simulink model "friction"  (R2017a)
settings: Solver=ode1  StartTime=0.0  StopTime=50  FixedStep=1e-3  RelTol=1e-3
values from neighbouring files (symbols this model uses):
  ctrl_mass = mass    (= 1)    [Script_Friction.m]
  ctrl_ts = 1e-3    (= 0.001)    [Script_Friction.m]
  Fapp = Fc/2    (= 1.5)    [Script_Friction.m]
  Fc = 2.4    [Script_Friction.m]
  Fs = 4.9    [Script_Friction.m]
  i = 6.7    [Script_Friction.m]
  kv = 40.101e-2    (= 0.40101)    [Script_Friction.m]
  m = 3.14    [Static_Identif.m]    (also in static_optim.m)
  mass = 8.1    [C_script_dyn_optimization.m]    (also in Script_Friction.m = 1; identify_dynamic_param.m)
  N = 100    [A_Static_Experiment.m]    (also in identify_static_param.m; obtain_sim_data.m = round(length(x) / 2); run_sim.m)
  sigma0 = 10e4    (= 100000)    [Script_Friction.m]
  sigma1 = 500    [Script_Friction.m]
  sigma2 = 0.1    [C_script_dyn_optimization.m]    (also in Script_Friction.m = 11.1)
  vs = 1.6e1    (= 16)    [Script_Friction.m]
  X = otim    [A_Static_Experiment.m]    (also in Static_Identif.m = X + 1.0 * V; identify_static_param.m; interval_definition.m = sprintf('Data from interval; static_optim.m = X + 1.0 * V)
undefined symbols (not defined in the file or in its folder): Y, Z
libraries: simulink x9, sm_lib x8, nesl_utility x5, fl_lib x2, checkpacklib x1, Multibody_Multiphysics_Lib x1
settings Model: Creator=jcmonteiro  LastModifiedBy=igricart
settings DataIOCC: ReturnWorkspaceOutputs=on  ReturnWorkspaceOutputsName=SDOSimTest_Log

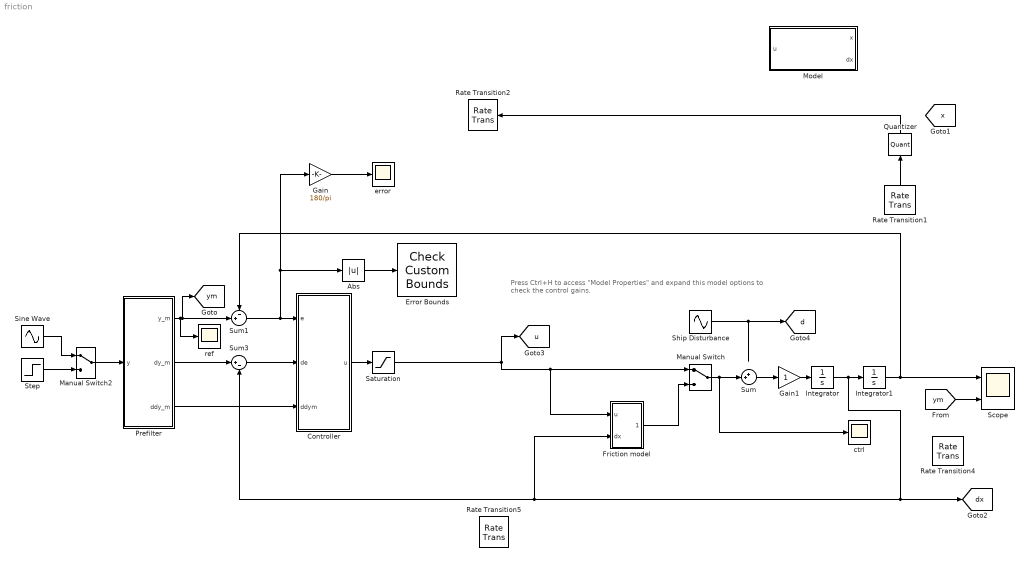
== system friction ==
  note: Press Ctrl+H to access "Model Properties" and expand this model options
      | to check the control gains.
  Abs : Abs
  Controller : Subsystem  mask{wn=0.5, damp=0.95, far=3}
      mask prompts: wn "Natural frequency"; damp "Damping"; far "Far pole"
      mask init:
      | Kd = far + 2*damp*wn;
      | Kp = wn*wn + 2*damp*wn*far;
      | Ki = far*wn*wn;
  Error Bounds : checkpacklib/Check Custom Bounds  InstantiateOnLoad=on  enabled=off  stopWhenAssertionFail=off  export=off  ViewDlgPos=[224 43 510 418]  OpenViewOnLoad=off  LaunchViewOnOpen=off  TimeUnits=seconds  EnableUpperBound=on  UpperBoundTimes=[0 1; 1 4; 4 20]  UpperBoundAmplitudes=[4e-3 4e-3; 2e-3 2e-3; 3.5e-4 3.5e-4];  EnableLowerBound=off  LowerBoundTimes=[]  LowerBoundAmplitudes=[]
  Friction model : Subsystem
  Gain : Gain  Gain=180/pi
  Gain1 : Gain
  Integrator : Integrator
  Integrator1 : Integrator
  Manual Switch : ManualSwitch
  Manual Switch2 : ManualSwitch
  Model : Subsystem
  Prefilter : Subsystem  mask{refmodel_wn=0.7, refmodel_eta=1}
      mask prompts: refmodel_wn "Natural Frequency"; refmodel_eta "Damping"
      mask init:
      | refmodel_eta = abs(refmodel_eta);
      | refmodel_eta = min(refmodel_eta, 1);
      | 
      | refmodel_wn = abs(refmodel_wn);
  Quantizer : Quantizer  QuantizationInterval=2*pi/2^18
  Rate Transition1 : RateTransition  OutPortSampleTime=daq_ts
  Rate Transition2 : RateTransition  OutPortSampleTime=ctrl_ts
  Rate Transition4 : RateTransition  OutPortSampleTime=daq_ts
  Rate Transition5 : RateTransition  OutPortSampleTime=ctrl_ts
  Saturation : Saturate  UpperLimit=20  LowerLimit=-20
  Scope : Scope  NumInputPorts=2
  Ship Disturbance : Sin  Frequency=2*pi/7  SampleTime=0
  Sine Wave : Sin  Amplitude=deg2rad(3)  Frequency=2*pi/8  SampleTime=ctrl_ts
  Step : Step  Time=0.1  After=deg2rad(10)  SampleTime=0
  Sum : Sum  Inputs=++|
  Sum1 : Sum  Inputs=-+|
  Sum3 : Sum  Inputs=|+-
  ctrl : Scope
  error : Scope
  ref : Scope
  tag scope: d=global, dx=global, u=global, x=global, ym=global
  wires:
  Manual Switch/1 -> Sum/2, ctrl/1
  Prefilter/1(y_m) -> ref/1, [ym], Sum1/2
  Prefilter/2(dy_m) -> Sum3/1
  [ym] -> Scope/2
  Controller/1(u) -> Saturation/1
  Sum3/1 -> Controller/2(de)
  Prefilter/3(ddy_m) -> Controller/3(ddym)
  Friction model/1(u_line) -> Manual Switch/2
  Abs/1 -> Error Bounds/1
  Sum1/1 -> Controller/1(e), Abs/1, Gain/1
  Rate Transition1/1 -> Quantizer/1
  Integrator1/1 -> Sum1/1, Scope/1
  Integrator/1 -> Sum3/2, Friction model/2(dx), [dx], Integrator1/1
  Ship Disturbance/1 -> [d]
  Gain/1 -> error/1
  Quantizer/1 -> Rate Transition2/1
  Saturation/1 -> Manual Switch/1, Friction model/1(u), [u]
  Manual Switch2/1 -> Prefilter/1(y)
  Sine Wave/1 -> Manual Switch2/1
  Step/1 -> Manual Switch2/2
  Sum/1 -> Gain1/1
  Gain1/1 -> Integrator/1
  ? -> [x]

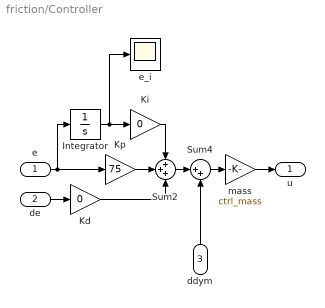
== system friction/Controller ==
  e : Inport  SampleTime=ctrl_ts
  de : Inport  Port=2  SampleTime=ctrl_ts
  ddym : Inport  Port=3  SampleTime=ctrl_ts
  Integrator : Integrator
  Kd : Gain  Gain=0
  Ki : Gain  Gain=0
  Kp : Gain  Gain=75
  Sum2 : Sum  Inputs=+++
  Sum4 : Sum  Inputs=|++
  e_i : Scope
  mass : Gain  Gain=ctrl_mass
  u : Outport  SampleTime=ctrl_ts
  wires:
  Integrator/1 -> e_i/1, Ki/1
  Sum4/1 -> mass/1
  Ki/1 -> Sum2/1
  de/1 -> Kd/1
  Kd/1 -> Sum2/3
  Kp/1 -> Sum2/2
  mass/1 -> u/1
  e/1 -> Integrator/1, Kp/1
  ddym/1 -> Sum4/2
  Sum2/1 -> Sum4/1

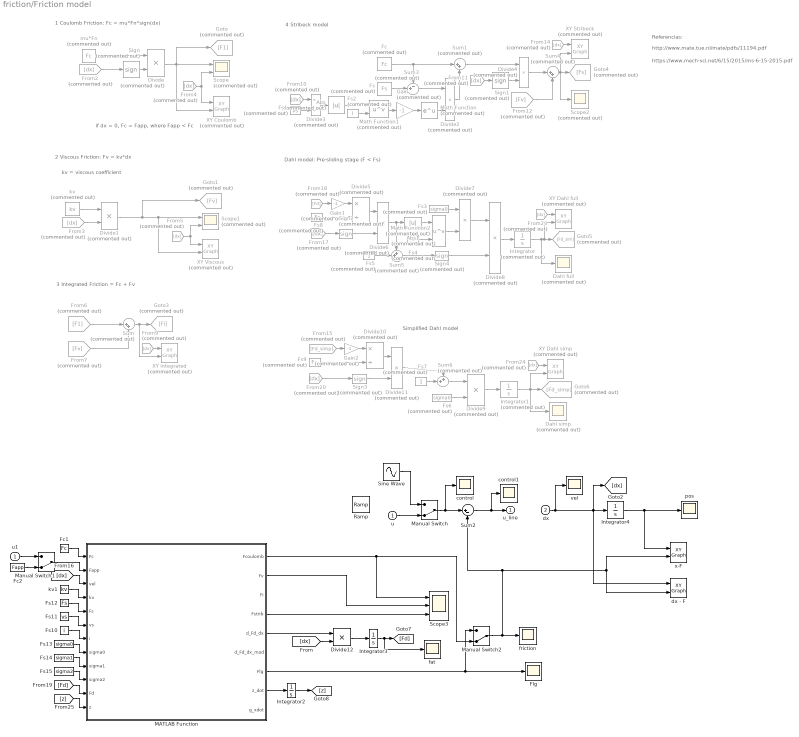
== system friction/Friction model ==
  note: Simplified Dahl model
  note: Dahl model: Pre-sliding stage (F < Fs)
  note: 4 Stribeck model
  note: 3 Integrated Friction = Fc + Fv
  note: if dx = 0, Fc = Fapp, where Fapp < Fc
  note: kv = viscous coefficient
  note: https://www.mech-sci.net/6/15/2015/ms-6-15-2015.pdf
  note: Referencias:
  note: http://www.mate.tue.nl/mate/pdfs/11194.pdf
  note: 1 Coulomb Friction: Fc = mu*Fn*sign(dx)
  note: 2 Viscous Friction: Fv = kv*dx
  u : Inport
  dx : Inport  Port=2
  Abs : Abs  Commented=on
  Abs1 : Abs  Commented=on
  Dahl full : Scope  Commented=on
  Dahl simp : Scope  Commented=on
  Divide{,1..2,4,6..9,11} (9 alike) : Product  Commented=on  Inputs=**
  Divide10 : Product  Commented=on  Inputs=*/
  Divide12 : Product  Inputs=**
  Divide3 : Product  Commented=on  Inputs=*/
  Divide5 : Product  Commented=on  Inputs=*/
  Fc : Constant  Commented=on  Value=Fc
  Fc1 : Constant  Value=Fc
  Fc2 : Constant  Value=Fapp
  Flg : Scope
  From{2..5,9..11,14,17,20,23..24} (12 alike) : From  Commented=on  GotoTag=dx
  From12 : From  Commented=on  GotoTag=Fv
  From15 : From  Commented=on  GotoTag=Fd_simp
  From18 : From  Commented=on  GotoTag=Fd
  From6 : From  Commented=on  GotoTag=F1
  From7 : From  Commented=on  GotoTag=Fv
  Fs : Constant  Commented=on  Value=Fs
  Fs1 : Constant  Commented=on  Value=vs
  Fs10 : Constant  Value=i
  Fs11 : Constant  Value=vs
  Fs12 : Constant  Value=Fs
  Fs13 : Constant  Value=sigma0
  Fs14 : Constant  Value=sigma1
  Fs15 : Constant  Value=sigma2
  Fs2 : Constant  Commented=on  Value=i
  Fs3 : Constant  Commented=on  Value=sigma0
  Fs4 : Constant  Commented=on  Value=i
  Fs5 : Constant  Commented=on
  Fs6 : Constant  Commented=on  Value=sigma0
  Fs7 : Constant  Commented=on
  Fs8 : Constant  Commented=on  Value=Fc
  Fs9 : Constant  Commented=on  Value=Fc
  Gain : Gain  Commented=on  Gain=-1
  Gain1 : Gain  Commented=on  Gain=-1
  Gain2 : Gain  Commented=on  Gain=-1
  Goto : Goto  Commented=on  GotoTag=F1
  Goto1 : Goto  Commented=on  GotoTag=Fv
  Goto3 : Goto  Commented=on  GotoTag=Fi
  Goto4 : Goto  Commented=on  GotoTag=Fs
  Goto5 : Goto  Commented=on  GotoTag=Fd_sim
  Goto6 : Goto  Commented=on  GotoTag=Fd_simp
  Integrator : Integrator  Commented=on  InitialCondition=Fc
  Integrator1 : Integrator  Commented=on  InitialCondition=Fc
  Integrator2 : Integrator
  Integrator3 : Integrator
  Integrator4 : Integrator
  MATLAB Function : MATLAB Function  TreatAsAtomicUnit=on
  Manual Switch : ManualSwitch  CurrentSetting=0
  Manual Switch1 : ManualSwitch  CurrentSetting=0
  Manual Switch2 : ManualSwitch  CurrentSetting=0
  Math Function : Math  Commented=on  SaturateOnIntegerOverflow=on
  Math Function1 : Math  Commented=on  Operator=pow  SaturateOnIntegerOverflow=on
  Math Function2 : Math  Commented=on  Operator=pow  SaturateOnIntegerOverflow=on
  Ramp : simulink/Sources/Ramp  slope=0.2  start=0  X0=0
  Scope : Scope  Commented=on  NumInputPorts=2
  Scope1 : Scope  Commented=on  NumInputPorts=2
  Scope2 : Scope  Commented=on
  Scope3 : Scope  NumInputPorts=3
  Sign{,1..4} (5 alike) : Signum  Commented=on
  Sine Wave : Sin  Amplitude=3  Frequency=2*pi/5  SampleTime=0
  Sum : Sum  Commented=on  Inputs=|++
  Sum1 : Sum  Commented=on  Inputs=|++
  Sum2 : Sum  Inputs=|+-
  Sum3 : Sum  Commented=on  Inputs=-+|
  Sum4 : Sum  Commented=on  Inputs=|++
  Sum5 : Sum  Commented=on  Inputs=++|
  Sum6 : Sum  Commented=on  Inputs=++|
  XY Coulomb : simulink/Sinks/XY Graph  Commented=on  xmin=-0.15  xmax=0.15  ymin=-15  ymax=15  st=-1
  XY Dahl full : simulink/Sinks/XY Graph  Commented=on  xmin=-0.2  xmax=0.2  ymin=0  ymax=5  st=-1
  XY Dahl simp : simulink/Sinks/XY Graph  Commented=on  xmin=-0.15  xmax=0.15  ymin=-15  ymax=15  st=-1
  XY Stribeck : simulink/Sinks/XY Graph  Commented=on  xmin=-0.15  xmax=0.15  ymin=-15  ymax=15  st=-1
  XY Viscous : simulink/Sinks/XY Graph  Commented=on  xmin=-0.15  xmax=0.15  ymin=-15  ymax=15  st=-1
  XY integrated : simulink/Sinks/XY Graph  Commented=on  xmin=-0.15  xmax=0.15  ymin=-15  ymax=15  st=-1
  control : Scope
  control1 : Scope
  dx - F : simulink/Sinks/XY Graph  xmin=-1  xmax=1  ymin=-10  ymax=5  st=-1
  fat : Scope
  friction : Scope
  kv : Constant  Commented=on  Value=kv
  kv1 : Constant  Value=kv
  mu*Fn : Constant  Commented=on  Value=Fc
  pos : Scope
  u1 : InportShadow
  vel : Scope
  x-F : simulink/Sinks/XY Graph  xmin=-0.01  xmax=0.01  ymin=-2.2  ymax=2.2  st=-1
  u_line : Outport
  wires:
  Sign/1 -> Divide/2
  mu*Fn/1 -> Divide/1
  Sum2/1 -> control1/1, u_line/1
  kv/1 -> Divide1/1
  dx/1 -> vel/1, dx - F/1, [dx], Integrator4/1
  From2/1 -> Sign/1
  Divide1/1 -> XY Viscous/2, Scope1/1, Goto1/1
  From3/1 -> Divide1/2
  Divide/1 -> XY Coulomb/2, Goto/1, Scope/1
  From4/1 -> Scope/2, XY Coulomb/1
  From5/1 -> XY Viscous/1, Scope1/2
  From6/1 -> Sum/1
  From7/1 -> Sum/2
  Sum/1 -> XY integrated/2, Goto3/1
  From9/1 -> XY integrated/1
  Fc/1 -> Sum3/1, Sum1/1
  Fs/1 -> Sum3/2
  Sum3/1 -> Divide2/1
  Math Function/1 -> Divide2/2
  From10/1 -> Divide3/1
  Fs1/1 -> Divide3/2
  Divide3/1 -> Abs/1
  Math Function1/1 -> Gain/1
  Fs2/1 -> Math Function1/2
  Gain/1 -> Math Function/1
  Abs/1 -> Math Function1/1
  Divide2/1 -> Sum1/2
  Sign1/1 -> Divide4/2
  From11/1 -> Sign1/1
  Sum1/1 -> Divide4/1
  Divide4/1 -> Sum4/1
  From12/1 -> Sum4/2
  Sum4/1 -> Scope2/1, XY Stribeck/2, Goto4/1
  From14/1 -> XY Stribeck/1
  From17/1 -> Sign2/1
  Fs8/1 -> Divide5/2
  From18/1 -> Gain1/1
  Gain1/1 -> Divide5/1
  Divide5/1 -> Divide6/1
  Sign2/1 -> Divide6/2
  Divide6/1 -> Sum5/1, Abs1/1
  Fs4/1 -> Math Function2/2
  Abs1/1 -> Math Function2/1
  Math Function2/1 -> Divide7/2
  Fs3/1 -> Divide7/1
  Divide7/1 -> Divide8/1
  Sum5/1 -> Sign4/1
  Divide8/1 -> Integrator/1
  Fs6/1 -> Divide9/2
  Fs5/1 -> Sum5/2
  Divide9/1 -> Integrator1/1
  Fs7/1 -> Sum6/2
  Sum6/1 -> Divide9/1
  Divide11/1 -> Sum6/1
  Sign3/1 -> Divide11/2
  Divide10/1 -> Divide11/1
  Gain2/1 -> Divide10/1
  From15/1 -> Gain2/1
  Fs9/1 -> Divide10/2
  From20/1 -> Sign3/1
  Integrator/1 -> Dahl full/1, XY Dahl full/2, Goto5/1
  From23/1 -> XY Dahl full/1
  From24/1 -> XY Dahl simp/1
  Integrator1/1 -> Dahl simp/1, XY Dahl simp/2, Goto6/1
  Sign4/1 -> Divide8/2
  [dx] -> MATLAB Function/3(vel)
  Fs10/1 -> MATLAB Function/7(i)
  Fs11/1 -> MATLAB Function/6(vs)
  Fs12/1 -> MATLAB Function/5(Fs)
  kv1/1 -> MATLAB Function/4(kv)
  Fc1/1 -> MATLAB Function/1(Fc)
  MATLAB Function/4(Fstrib) -> Scope3/3
  Fs13/1 -> MATLAB Function/8(sigma0)
  Integrator3/1 -> fat/1, [Fd]
  [Fd] -> MATLAB Function/11(Fd)
  Integrator2/1 -> [z]
  MATLAB Function/8(z_dot) -> Integrator2/1
  Fs14/1 -> MATLAB Function/9(sigma1)
  Fs15/1 -> MATLAB Function/10(sigma2)
  [z] -> MATLAB Function/12(z)
  MATLAB Function/7(Flg) -> Manual Switch2/1, Flg/1
  MATLAB Function/5(d_Fd_dx) -> Divide12/1
  Divide12/1 -> Integrator3/1
  [dx] -> Divide12/2
  Manual Switch/1 -> control/1, Sum2/1
  u/1 -> Manual Switch/2
  MATLAB Function/2(Fv) -> Scope3/2
  MATLAB Function/1(Fcoulomb) -> Manual Switch2/2, Scope3/1
  Integrator4/1 -> x-F/1, pos/1
  Manual Switch1/1 -> MATLAB Function/2(Fapp)
  Fc2/1 -> Manual Switch1/2
  u1/1 -> Manual Switch1/1
  Manual Switch2/1 -> friction/1, x-F/2, dx - F/2, Sum2/2
  Sine Wave/1 -> Manual Switch/1

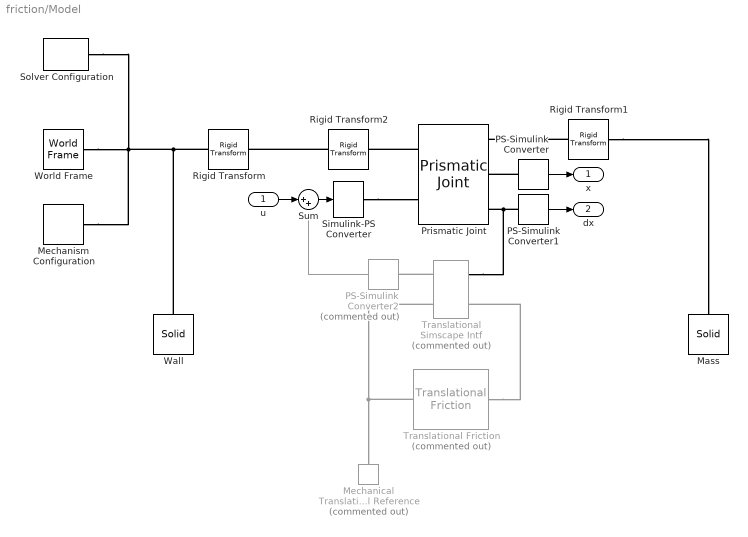
== system friction/Model ==
  u : Inport
  Mass : sm_lib/Body Elements/Solid  InertiaType=CalculateFromGeometry  Mass=mass  MassUnits=kg  CenterOfMass=[0 0 0]  CenterOfMassUnits=m  MomentsOfInertia=[1 1 1]  MomentsOfInertiaUnits=kg*m^2  ProductsOfInertia=[1 1 1]  ProductsOfInertiaUnits=kg*m^2  DensityBased=off  Density=mass * 1000  DensityUnits=kg/m^3  DoExposeReferenceFrame=on  SerializedFrames=<Frames/>  GraphicType=FromGeometry  MarkerShape=Sphere  MarkerSize=10  GraphicVisPropType=SimpleVisualProperties  GraphicDiffuseColor=[0.5 0.5 0.5]  GraphicSpecularColor=[0.5 0.5 0.5 1.0]  GraphicAmbientColor=[0.15 0.15 0.15 1.0]  GraphicEmissiveColor=[0.0 0.0 0.0 1.0]  GraphicShininess=75  GraphicOpacity=1.0  GeometryShape=Brick  RectangleSize=[1 1]  RectangleSizeUnits=m  BrickDimensions=[10 10 10]  BrickDimensionUnits=cm  CylinderRadius=1  CylinderRadiusUnits=m  CylinderLength=1  CylinderLengthUnits=m  SphereRadius=1  SphereRadiusUnits=m  EllipsoidRadii=[1 1 1]  EllipsoidRadiiUnits=m  ExtrusionCrossSection=[1 1; -1 1; -1 -1; 1 -1]  ExtrusionCrossSectionUnits=m  ExtrusionLength=1  ExtrusionLengthUnits=m  PolygonNumSides=3  PolygonOuterRadius=1  PolygonOuterRadiusUnits=m  ExtGeomFileType=STEP  ExtGeomFileUnits=m  RevolutionCrossSection=[1 1; 1 -1; 2 -1; 2 1]  RevolutionCrossSectionUnits=m  RevolutionExtent=Full  RevolutionAngle=180  RevolutionAngleUnits=deg
  Mechanical Translational Reference : fl_lib/Mechanical/Translational Elements/Mechanical Translational Reference  Commented=on
  Mechanism Configuration : sm_lib/Utilities/Mechanism Configuration  UniformGravity=Constant  GravityVector=[0 0 0]  GravityUnits=m/s^2  LinearizationDelta=0.001
  PS-Simulink Converter : nesl_utility/PS-Simulink Converter  PhysicalDomain=network_engine_domain  SubClassName=ps_output  LeftPortType=input  RightPortType=output  PseudoPeriodic=off  Frequencies=[]  Unit=1  AffineConversion=off
  PS-Simulink Converter1 : nesl_utility/PS-Simulink Converter  PhysicalDomain=network_engine_domain  SubClassName=ps_output  LeftPortType=input  RightPortType=output  PseudoPeriodic=off  Frequencies=[]  Unit=1  AffineConversion=off
  PS-Simulink Converter2 : nesl_utility/PS-Simulink Converter  Commented=on  PhysicalDomain=network_engine_domain  SubClassName=ps_output  LeftPortType=input  RightPortType=output  PseudoPeriodic=off  Frequencies=[]  Unit=N  AffineConversion=off
  Prismatic Joint : sm_lib/Joints/Prismatic Joint  SenseConstraintForce=off  SenseConstraintForceX=off  SenseConstraintForceY=off  SenseConstraintForceZ=off  SenseConstraintTorque=off  SenseConstraintTorqueX=off  SenseConstraintTorqueY=off  SenseConstraintTorqueZ=off  SenseTotalForce=off  SenseTotalForceX=off  SenseTotalForceY=off  SenseTotalForceZ=off  SenseTotalTorque=off  SenseTotalTorqueX=off  SenseTotalTorqueY=off  SenseTotalTorqueZ=off  CompositeWrenchDir=FollowerOnBase  CompositeWrenchFrame=BaseFrame  EquilibriumPosition=0  EquilibriumPositionUnits=m  SpringStiffness=0  SpringStiffnessUnits=N/m  DampingCoefficient=0  DampingCoefficientUnits=N/(m/s)  TorqueActuationMode=InputTorque  MotionActuationMode=ComputedMotion  SensePosition=on  SenseVelocity=on  SenseAcceleration=off  SenseTorqueForce=off  PositionTargetSpecify=off  PositionTargetPriority=High  PositionTargetValue=10  PositionTargetValueUnits=cm  VelocityTargetSpecify=off  VelocityTargetPriority=High  VelocityTargetValue=0  VelocityTargetValueUnits=m/s
  Rigid Transform : sm_lib/Frames and Transforms/Rigid Transform  TranslationMethod=StandardAxis  TranslationStandardOffset=11  TranslationLengthUnit=cm  TranslationStandardAxis=+X  TranslationCartesianOffset=[0 0 0]  TranslationROffset=0  TranslationROffsetUnits=m  TranslationZOffset=0  TranslationZOffsetUnits=m  TranslationThetaOffset=0  TranslationThetaOffsetUnits=deg  RotationMethod=None  RotationAngleUnits=deg  RotationStandardAxis=+Z  RotationAngle=0.0  RotationArbitraryAxis=[0 0 1]  FollAlignAxisA=+X  BaseAlignAxisA=+Y  FollAlignAxisB=+Y  BaseAlignAxisB=+Z  RotationSequenceAxes=FollowerAxes  RotationSequence=XYX  RotationSequenceAngles=[0 0 0]  RotationSequenceAnglesUnits=deg  RotationMatrix=[1 0 0; 0 1 0; 0 0 1]
  Rigid Transform1 : sm_lib/Frames and Transforms/Rigid Transform  TranslationMethod=None  TranslationStandardOffset=11  TranslationLengthUnit=cm  TranslationStandardAxis=+X  TranslationCartesianOffset=[0 0 0]  TranslationROffset=0  TranslationROffsetUnits=m  TranslationZOffset=0  TranslationZOffsetUnits=m  TranslationThetaOffset=0  TranslationThetaOffsetUnits=deg  RotationMethod=AlignedAxes  RotationAngleUnits=deg  RotationStandardAxis=+Z  RotationAngle=0.0  RotationArbitraryAxis=[0 0 1]  FollAlignAxisA=+X  BaseAlignAxisA=+Z  FollAlignAxisB=+Y  BaseAlignAxisB=+X  RotationSequenceAxes=FollowerAxes  RotationSequence=XYX  RotationSequenceAngles=[0 0 0]  RotationSequenceAnglesUnits=deg  RotationMatrix=[1 0 0; 0 1 0; 0 0 1]
  Rigid Transform2 : sm_lib/Frames and Transforms/Rigid Transform  TranslationMethod=None  TranslationStandardOffset=11  TranslationLengthUnit=cm  TranslationStandardAxis=+X  TranslationCartesianOffset=[0 0 0]  TranslationROffset=0  TranslationROffsetUnits=m  TranslationZOffset=0  TranslationZOffsetUnits=m  TranslationThetaOffset=0  TranslationThetaOffsetUnits=deg  RotationMethod=AlignedAxes  RotationAngleUnits=deg  RotationStandardAxis=+Z  RotationAngle=0.0  RotationArbitraryAxis=[0 0 1]  FollAlignAxisA=+Z  BaseAlignAxisA=+X  FollAlignAxisB=+X  BaseAlignAxisB=+Y  RotationSequenceAxes=FollowerAxes  RotationSequence=XYX  RotationSequenceAngles=[0 0 0]  RotationSequenceAnglesUnits=deg  RotationMatrix=[1 0 0; 0 1 0; 0 0 1]
  Simulink-PS Converter : nesl_utility/Simulink-PS Converter  PhysicalDomain=network_engine_domain  SubClassName=ps_input  LeftPortType=input  RightPortType=output  PseudoPeriodic=off  Frequencies=[]  NoiseDistribution=none  NoiseParameters=[]  Unit=N  AffineConversion=off  FilteringAndDerivatives=zero  SimscapeFilterOrder=1  InputFilterTimeConstant=0.001  UdotUserProvided=1
  Solver Configuration : nesl_utility/Solver Configuration  PhysicalDomain=network_engine_domain  SubClassName=solver  LeftPortType=input  RightPortType=generic  Accelerate=off  Tones=[]  Harmonics=[]  SimulateNoise=off  Profile=off  UseLocalSampling=off  EnableSwitchedLinearOptims=on  FrequencyDomain=off  UseCCode=off  RelTol=0.001  AbsTol=1e-06  MinStep=1e-09  ToWorkspace=off  RevertToSquareIcSolve=off  NumHomotopyIterations=100  PhasorMode=off  PhasorModeNumHarmonics=1  OverrideAbsTol=off  DoDC=on  ResidualTolerance=1e-09  UseLocalSolver=off  LocalSolverChoice=NE_BACKWARD_EULER_ADVANCER  LocalSolverSampleTime=0.001  DoFixedCost=off  MaxNonlinIter=3  MaxModeIter=2  LinearAlgebra=Sparse  DelaysMemoryBudget=1024  AutomaticFiltering=on  FilteringTimeConstant=0.001
  Sum : Sum  Inputs=|++
  Translational Friction : fl_lib/Mechanical/Translational Elements/Translational Friction  Commented=on  brkwy_frc=0.8 N  brkwy_vel=deg2rad(0.5) m/s  Col_frc=0.7 N  visc_coef=0 N/(m/s)  v_specify=off  v_priority=High  v=0 m/s  v_nominal_specify=off  v_nominal_unit=m/s  v_nominal_value=1  f_specify=off  f_priority=None  f=0 N  f_nominal_specify=off  f_nominal_unit=N  f_nominal_value=1
      settings: SourceProductName=Simscape  SourceProductBaseCode=SS
  Translational Simscape Intf : Multibody_Multiphysics_Lib/Interfaces/Translational Simscape Intf  Commented=on
      settings: SourceProductName=Simscape Multibody Multiphysics Library
  Wall : sm_lib/Body Elements/Solid  InertiaType=CalculateFromGeometry  Mass=1  MassUnits=kg  CenterOfMass=[0 0 0]  CenterOfMassUnits=m  MomentsOfInertia=[1 1 1]  MomentsOfInertiaUnits=kg*m^2  ProductsOfInertia=[1 1 1]  ProductsOfInertiaUnits=kg*m^2  DensityBased=on  Density=1000  DensityUnits=kg/m^3  DoExposeReferenceFrame=on  SerializedFrames=<Frames/>  GraphicType=FromGeometry  MarkerShape=Sphere  MarkerSize=10  GraphicVisPropType=SimpleVisualProperties  GraphicDiffuseColor=[0.5 0.5 0.5]  GraphicSpecularColor=[0.5 0.5 0.5 1.0]  GraphicAmbientColor=[0.15 0.15 0.15 1.0]  GraphicEmissiveColor=[0.0 0.0 0.0 1.0]  GraphicShininess=75  GraphicOpacity=1.0  GeometryShape=Brick  RectangleSize=[1 1]  RectangleSizeUnits=m  BrickDimensions=[1 100 100]  BrickDimensionUnits=cm  CylinderRadius=1  CylinderRadiusUnits=m  CylinderLength=1  CylinderLengthUnits=m  SphereRadius=1  SphereRadiusUnits=m  EllipsoidRadii=[1 1 1]  EllipsoidRadiiUnits=m  ExtrusionCrossSection=[1 1; -1 1; -1 -1; 1 -1]  ExtrusionCrossSectionUnits=m  ExtrusionLength=1  ExtrusionLengthUnits=m  PolygonNumSides=3  PolygonOuterRadius=1  PolygonOuterRadiusUnits=m  ExtGeomFileType=STEP  ExtGeomFileUnits=m  RevolutionCrossSection=[1 1; 1 -1; 2 -1; 2 1]  RevolutionCrossSectionUnits=m  RevolutionExtent=Full  RevolutionAngle=180  RevolutionAngleUnits=deg
  World Frame : sm_lib/Frames and Transforms/World Frame
  x : Outport
  dx : Outport  Port=2
  wires:
  u/1 -> Sum/1
  PS-Simulink Converter/1 -> x/1
  PS-Simulink Converter1/1 -> dx/1
  PS-Simulink Converter2/1 -> ?
  Sum/1 -> Simulink-PS Converter/1
  connections:
  Simulink-PS Converter/RConn1 -- Prismatic Joint/LConn2
  Wall/RConn1 -- Rigid Transform/LConn1 -- Solver Configuration/RConn1 -- Mechanism Configuration/RConn1 -- World Frame/RConn1
  Rigid Transform2/LConn1 -- Rigid Transform/RConn1
  Rigid Transform1/RConn1 -- Mass/RConn1
  Rigid Transform1/LConn1 -- Prismatic Joint/RConn1
  Prismatic Joint/LConn1 -- Rigid Transform2/RConn1
  PS-Simulink Converter/LConn1 -- Prismatic Joint/RConn2
  PS-Simulink Converter1/LConn1 -- Translational Simscape Intf/RConn1 -- Prismatic Joint/RConn3
  Translational Friction/RConn1 -- Mechanical Translational Reference/LConn1 -- Translational Simscape Intf/LConn2
  Translational Friction/LConn1 -- Translational Simscape Intf/RConn2
  Translational Simscape Intf/LConn1 -- PS-Simulink Converter2/LConn1

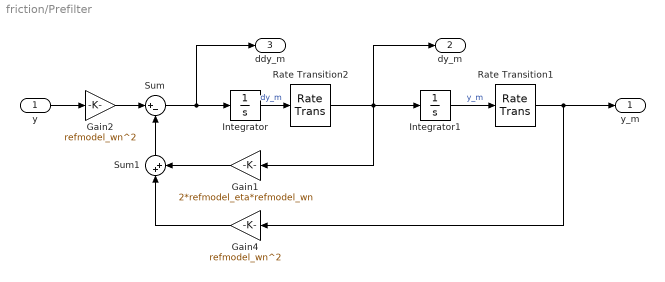
== system friction/Prefilter ==
  y : Inport
  Gain1 : Gain  Gain=2*refmodel_eta*refmodel_wn
  Gain2 : Gain  Gain=refmodel_wn^2
  Gain4 : Gain  Gain=refmodel_wn^2
  Integrator : Integrator
  Integrator1 : Integrator
  Rate Transition1 : RateTransition  OutPortSampleTime=ctrl_ts
  Rate Transition2 : RateTransition  OutPortSampleTime=ctrl_ts
  Sum : Sum  Inputs=|+-
  Sum1 : Sum  Inputs=|++
  y_m : Outport
  dy_m : Outport  Port=2
  ddy_m : Outport  Port=3
  wires:
  Sum/1 -> Integrator/1, ddy_m/1
  Integrator/1 -> Rate Transition2/1  "dy_m"
  Integrator1/1 -> Rate Transition1/1  "y_m"
  Gain4/1 -> Sum1/1
  Gain2/1 -> Sum/1
  y/1 -> Gain2/1
  Gain1/1 -> Sum1/2
  Sum1/1 -> Sum/2
  Rate Transition2/1 -> Gain1/1, Integrator1/1, dy_m/1
  Rate Transition1/1 -> y_m/1, Gain4/1

== matlab function friction/Friction model/MATLAB Function ==
  data: Fcoulomb output; Fc input; Fapp input; vel input; kv input; Fs input; vs input; i input; sigma0 input; sigma1 input; sigma2 input; Fv output; Fi output; Fstrib output; Fd input; d_Fd_dx output; d_Fd_dx_mod output; Flg output; z_dot output; z input; g_xdot output
%% Function with friction models

function [Fcoulomb ,Fv ,Fi ,Fstrib ,d_Fd_dx ,d_Fd_dx_mod ,Flg ,z_dot,g_xdot] = friction(Fc ,Fapp ,vel ,kv ,Fs ,vs ,i ,sigma0 ,sigma1 ,sigma2 ,Fd ,z )

%% Coulomb Friction and Viscous Friction
if (vel ~= 0)
   Fcoulomb = Fc*sign(vel);
   Fv = kv*vel;
else
    Fcoulomb = Fapp;
    Fv = Fapp;
end

%% Integrated Coulomb Friction and Viscous Friction with friction force
% transition
if (vel >= 0)
    Fi = min(Fc,Fv);
else
    Fi = max(-Fc,Fv);
end

%% Stribeck model
Fstrib = (Fc + (Fs - Fc) * exp(-(abs(vel/vs))^i)) * sign(vel) + Fv;

%% Dahl Model - Pre-sliding (Fd < Fs)
d_Fd_dx = sigma0 * (abs(1 - Fd/Fc * sign(vel)))^i * sign(1 - Fd / Fc * sign(vel));

%Simplified model where i = 1
d_Fd_dx_mod = sigma0 * (1 - Fd/Fc * sign(vel));

d_Fd_dx_mod = 0;
%% LeGru model
% Alpeter dc thesis
% Normally i  =  2
% g_xdot = Fc + (Fs - Fc) * exp(-(abs(vel/vs))^i);
% z_dot = vel - sigma0 * vel * z / g_xdot;
% Flg = sigma0 * z + sigma1 * z_dot + sigma2 * vel;

% Olsson paper
g_xdot = Fc + (Fs - Fc) * exp(-i*abs(vel));
z_dot = vel - sigma0 * abs(vel) * z / g_xdot;
Flg = sigma0 * z + sigma1 * z_dot + sigma2 * vel;
